simulink model "posMeas_stream"  (R2016a)
settings: Solver=FixedStepDiscrete  SolverMode=SingleTasking  StartTime=0.0  StopTime=inf  FixedStep=1/50  RelTol=1e-3
libraries: sldrtlib x1, dspvision x1, dspnetwork x1
settings Model: Creator=gurtnmar  LastModifiedBy=marti
settings DataIOCC: LimitDataPoints=on  SaveFormat=Array
settings OptimizationCC: BlockReduction=off  BooleanDataType=off
settings DebuggingCC: SaveWithParameterizedLinksMsg=none  UnderspecifiedInitializationDetection=Classic  MergeDetectMultiDrivingBlocksExec=none  SignalResolutionControl=TryResolveAllWithWarning
settings HardwareCC: ProdBitPerPointer=32  ProdLargestAtomicFloat=None  ProdIntDivRoundTo=Undefined  ProdEndianess=Unspecified  ProdWordSize=32  ProdHWDeviceType=32-bit Generic  TargetUnknown=on
settings ModelReferenceCC: PropagateSignalLabelsOutOfModel=off

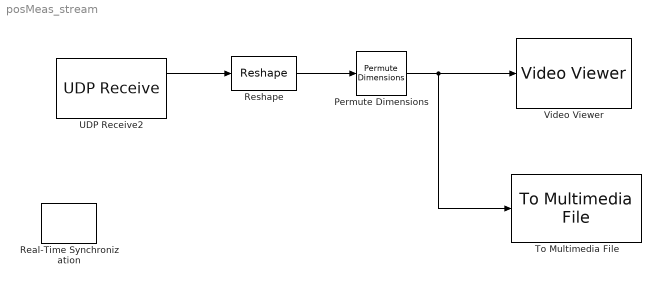
== system posMeas_stream ==
  Permute Dimensions : PermuteDimensions
  Real-Time Synchronization : sldrtlib/Real-Time Synchronization  SampleTime=1/50  MaxMissedTicks=10  ShowMissedTicks=off  YieldWhenWaiting=off
  Reshape : Reshape  OutputDimensionality=Customize  OutputDimensions=[(2*64), (2*64)]
  To Multimedia File : dspvision/To Multimedia File  outputFilename=output.avi  streamSelection=Video only  videoCompressor=None (uncompressed)  audioCompressor=None (uncompressed)  imagePorts=One multidimensional signal  fileType=AVI  audioDatatype=Determine from input data type  fourcc=RGB  videoQuality=75  mj2000CompFactor=10
  UDP Receive2 : dspnetwork/UDP Receive  localURL='0.0.0.0'  localPort=9899  remoteURL='0.0.0.0'  remotePort=-1  recvBufferSize=(2*64)^2  dims=(2*64)^2  signalDatatype=uint8  isVarSize=off  showBlockingTime=on  blockingTime=5  sampletime=1/50  blockPlatform=HOST
  Video Viewer : VideoViewer  FigPos=[49 1897 739 485]
  wires:
  UDP Receive2/1 -> Reshape/1
  Reshape/1 -> Permute Dimensions/1
  Permute Dimensions/1 -> To Multimedia File/1, Video Viewer/1
